simulink model "test_bu01_2018b"  (R2018b)
settings: Solver=FixedStepAuto  StartTime=0.0  StopTime=10  FixedStep=0.02  RelTol=1e-3
model workspace (MAT data in the model file):
  Ixx = 0.8
  Iyy = 2.075
  Izz = 1.25
  K = 0.75
  Mass = 11.5
  b = 0
libraries: simulink x10, aerolibutil x6, vrlib x4, sharedtransform x4, sharedutil x3, shared6dof x1
(part 4 of 4)

== system test_bu01_2018b/bu01_model/动力系统模型/Motor1_TM_P/TM1654P /螺旋桨模型/螺旋桨气动/计算螺旋桨气动系数/计算Ctz ==
  Miu : Inport
  Lumda : Inport  Port=2
  Add2 : Sum  Inputs=++-+-
  Add3 : Sum  Inputs=++-+
  Constant3 : Constant  Value=0.0651
  Constant4 : Constant  Value=0.0845
  Gain10 : Gain  Gain=0.0583
  Gain11 : Gain  Gain=0.3529
  Gain6 : Gain  Gain=0.0579
  Gain7 : Gain  Gain=0.0066
  Gain8 : Gain  Gain=-0.2325
  Gain9 : Gain  Gain=0.1346
  Lumda1 : InportShadow  Port=2
  Multiply2 : Product
  Square3 : Math  Operator=square  SaturateOnIntegerOverflow=on
  Square4 : Math  Operator=square  SaturateOnIntegerOverflow=on
  Square5 : Math  Operator=square  SaturateOnIntegerOverflow=on
  Ctz : Outport
  wires:
  Gain7/1 -> Add3/3
  Gain6/1 -> Add3/2
  Multiply2/1 -> Add3/4
  Add3/1 -> Ctz/1  "Ctz"
  Miu/1 -> Square4/1, Gain6/1, Square3/1, Gain8/1
  Lumda/1 -> Square5/1, Gain10/1
  Constant3/1 -> Add3/1
  Add2/1 -> Multiply2/2
  Square4/1 -> Gain9/1
  Constant4/1 -> Add2/3
  Gain9/1 -> Add2/2
  Square5/1 -> Gain11/1
  Gain11/1 -> Add2/5
  Gain8/1 -> Add2/1
  Square3/1 -> Gain7/1
  Gain10/1 -> Add2/4
  Lumda1/1 -> Multiply2/1

== system test_bu01_2018b/bu01_model/动力系统模型/Motor2_TM_N/TM1654N /螺旋桨模型/螺旋桨气动/计算螺旋桨气动系数/计算Cmx ==
  Miu : Inport
  Lumda : Inport  Port=2
  Add : Sum  Inputs=++--
  Constant : Constant  Value=0.0101
  Gain : Gain  Gain=0.0041
  Gain1 : Gain  Gain=0.009
  Gain2 : Gain  Gain=0.0032
  Multiply : Product
  Square : Math  Operator=square  SaturateOnIntegerOverflow=on
  Cmx : Outport
  wires:
  Multiply/1 -> Cmx/1  "Cmx"
  Lumda/1 -> Square/1, Gain1/1
  Gain2/1 -> Add/4
  Square/1 -> Gain2/1
  Gain/1 -> Add/2
  Constant/1 -> Add/1
  Miu/1 -> Multiply/1, Gain/1
  Gain1/1 -> Add/3
  Add/1 -> Multiply/2

== system test_bu01_2018b/bu01_model/动力系统模型/Motor2_TM_N/TM1654N /螺旋桨模型/螺旋桨气动/计算螺旋桨气动系数/计算Cmy ==
  Miu : Inport
  Lumda : Inport  Port=2
  Add1 : Sum  Inputs=++--
  Constant1 : Constant  Value=0.0101
  Gain1 : Gain  Gain=0.0041
  Gain3 : Gain  Gain=0.009
  Gain4 : Gain  Gain=0.0032
  Multiply1 : Product
  Square2 : Math  Operator=square  SaturateOnIntegerOverflow=on
  Cmy : Outport
  wires:
  Miu/1 -> Multiply1/1, Gain1/1
  Constant1/1 -> Add1/1
  Add1/1 -> Multiply1/2
  Gain4/1 -> Add1/4
  Square2/1 -> Gain4/1
  Lumda/1 -> Square2/1, Gain3/1
  Gain3/1 -> Add1/3
  Multiply1/1 -> Cmy/1  "Cmy"
  Gain1/1 -> Add1/2

== system test_bu01_2018b/bu01_model/动力系统模型/Motor2_TM_N/TM1654N /螺旋桨模型/螺旋桨气动/计算螺旋桨气动系数/计算Cmz ==
  Miu : Inport
  Lumda : Inport  Port=2
  Add2 : Sum  Inputs=+-+--
  Add3 : Sum  Inputs=+-++
  Constant3 : Constant  Value=0.0036
  Constant4 : Constant  Value=0.0023
  Gain10 : Gain  Gain=0.0105
  Gain11 : Gain  Gain=0.0078
  Gain6 : Gain  Gain=0.0006554
  Gain7 : Gain  Gain=0.00080732
  Gain8 : Gain  Gain=0.006
  Gain9 : Gain  Gain=0.0043
  Lumda1 : InportShadow  Port=2
  Multiply2 : Product
  Square3 : Math  Operator=square  SaturateOnIntegerOverflow=on
  Square4 : Math  Operator=square  SaturateOnIntegerOverflow=on
  Square5 : Math  Operator=square  SaturateOnIntegerOverflow=on
  Cmz : Outport
  wires:
  Lumda1/1 -> Multiply2/1
  Gain10/1 -> Add2/4
  Square3/1 -> Gain7/1
  Gain8/1 -> Add2/1
  Gain11/1 -> Add2/5
  Square5/1 -> Gain11/1
  Gain9/1 -> Add2/2
  Constant4/1 -> Add2/3
  Square4/1 -> Gain9/1
  Add2/1 -> Multiply2/2
  Constant3/1 -> Add3/1
  Lumda/1 -> Gain10/1, Square5/1
  Miu/1 -> Gain6/1, Square3/1, Square4/1, Gain8/1
  Add3/1 -> Cmz/1  "Cmz"
  Multiply2/1 -> Add3/4
  Gain6/1 -> Add3/2
  Gain7/1 -> Add3/3

== system test_bu01_2018b/bu01_model/动力系统模型/Motor2_TM_N/TM1654N /螺旋桨模型/螺旋桨气动/计算螺旋桨气动系数/计算Ctx ==
  Miu : Inport
  Lumda : Inport  Port=2
  Add : Sum  Inputs=++-+
  Constant : Constant  Value=-0.0074
  Gain : Gain  Gain=0.00051704
  Gain1 : Gain  Gain=0.0073
  Gain2 : Gain  Gain=0.018
  Multiply : Product
  Square : Math  Operator=square  SaturateOnIntegerOverflow=on
  Ctx : Outport
  wires:
  Add/1 -> Multiply/2
  Gain1/1 -> Add/3
  Miu/1 -> Multiply/1, Gain/1
  Constant/1 -> Add/1
  Gain/1 -> Add/2
  Square/1 -> Gain2/1
  Gain2/1 -> Add/4
  Lumda/1 -> Square/1, Gain1/1
  Multiply/1 -> Ctx/1  "Ctx"

== system test_bu01_2018b/bu01_model/动力系统模型/Motor2_TM_N/TM1654N /螺旋桨模型/螺旋桨气动/计算螺旋桨气动系数/计算Cty ==
  Miu : Inport
  Lumda : Inport  Port=2
  Add1 : Sum  Inputs=+++-
  Constant : Constant  Value=3
  Constant1 : Constant  Value=-0.002  OutDataTypeStr=double
  Gain3 : Gain  Gain=0.0103
  Gain4 : Gain  Gain=0.0168
  Gain5 : Gain  Gain=0.0897
  Multiply1 : Product
  Power : Math  Operator=pow  SaturateOnIntegerOverflow=on
  Square2 : Math  Operator=square  SaturateOnIntegerOverflow=on
  Cty : Outport
  wires:
  Gain5/1 -> Add1/4
  Multiply1/1 -> Cty/1  "Cty"
  Gain3/1 -> Add1/2
  Lumda/1 -> Power/1, Square2/1, Gain3/1
  Square2/1 -> Gain4/1
  Constant/1 -> Power/2
  Gain4/1 -> Add1/3
  Add1/1 -> Multiply1/2
  Constant1/1 -> Add1/1
  Power/1 -> Gain5/1
  Miu/1 -> Multiply1/1

== system test_bu01_2018b/bu01_model/动力系统模型/Motor2_TM_N/TM1654N /螺旋桨模型/螺旋桨气动/计算螺旋桨气动系数/计算Ctz ==
  Miu : Inport
  Lumda : Inport  Port=2
  Add2 : Sum  Inputs=++-+-
  Add3 : Sum  Inputs=++-+
  Constant3 : Constant  Value=0.0651
  Constant4 : Constant  Value=0.0845
  Gain10 : Gain  Gain=0.0583
  Gain11 : Gain  Gain=0.3529
  Gain6 : Gain  Gain=0.0579
  Gain7 : Gain  Gain=0.0066
  Gain8 : Gain  Gain=-0.2325
  Gain9 : Gain  Gain=0.1346
  Lumda1 : InportShadow  Port=2
  Multiply2 : Product
  Square3 : Math  Operator=square  SaturateOnIntegerOverflow=on
  Square4 : Math  Operator=square  SaturateOnIntegerOverflow=on
  Square5 : Math  Operator=square  SaturateOnIntegerOverflow=on
  Ctz : Outport
  wires:
  Gain7/1 -> Add3/3
  Gain6/1 -> Add3/2
  Multiply2/1 -> Add3/4
  Add3/1 -> Ctz/1  "Ctz"
  Miu/1 -> Gain8/1, Square4/1, Square3/1, Gain6/1
  Lumda/1 -> Square5/1, Gain10/1
  Constant3/1 -> Add3/1
  Add2/1 -> Multiply2/2
  Square4/1 -> Gain9/1
  Constant4/1 -> Add2/3
  Gain9/1 -> Add2/2
  Square5/1 -> Gain11/1
  Gain11/1 -> Add2/5
  Gain8/1 -> Add2/1
  Square3/1 -> Gain7/1
  Gain10/1 -> Add2/4
  Lumda1/1 -> Multiply2/1

== system test_bu01_2018b/bu01_model/动力系统模型/Motor3_TM_P/TM1654P /螺旋桨模型/螺旋桨气动/计算螺旋桨气动系数/计算Cmx ==
  Miu : Inport
  Lumda : Inport  Port=2
  Add : Sum  Inputs=++--
  Constant : Constant  Value=0.0101
  Gain : Gain  Gain=0.0041
  Gain1 : Gain  Gain=0.009
  Gain2 : Gain  Gain=0.0032
  Multiply : Product
  Square : Math  Operator=square  SaturateOnIntegerOverflow=on
  Cmx : Outport
  wires:
  Multiply/1 -> Cmx/1  "Cmx"
  Lumda/1 -> Square/1, Gain1/1
  Gain2/1 -> Add/4
  Square/1 -> Gain2/1
  Gain/1 -> Add/2
  Constant/1 -> Add/1
  Miu/1 -> Gain/1, Multiply/1
  Gain1/1 -> Add/3
  Add/1 -> Multiply/2

== system test_bu01_2018b/bu01_model/动力系统模型/Motor3_TM_P/TM1654P /螺旋桨模型/螺旋桨气动/计算螺旋桨气动系数/计算Cmy ==
  Miu : Inport
  Lumda : Inport  Port=2
  Add1 : Sum  Inputs=++++-
  Constant : Constant  Value=3
  Constant1 : Constant  Value=-0.015
  Gain1 : Gain  Gain=0.0115
  Gain2 : Gain  Gain=0.1908
  Gain3 : Gain  Gain=0.0146
  Gain4 : Gain  Gain=0.0484
  Multiply1 : Product
  Power : Math  Operator=pow  SaturateOnIntegerOverflow=on
  Square2 : Math  Operator=square  SaturateOnIntegerOverflow=on
  Cmy : Outport
  wires:
  Gain2/1 -> Add1/5
  Power/1 -> Gain2/1
  Constant/1 -> Power/2
  Miu/1 -> Multiply1/1, Gain1/1
  Constant1/1 -> Add1/1
  Add1/1 -> Multiply1/2
  Gain4/1 -> Add1/4
  Square2/1 -> Gain4/1
  Lumda/1 -> Square2/1, Power/1, Gain3/1
  Gain3/1 -> Add1/3
  Multiply1/1 -> Cmy/1  "Cmy"
  Gain1/1 -> Add1/2

== system test_bu01_2018b/bu01_model/动力系统模型/Motor3_TM_P/TM1654P /螺旋桨模型/螺旋桨气动/计算螺旋桨气动系数/计算Cmz ==
  Miu : Inport
  Lumda : Inport  Port=2
  Add2 : Sum  Inputs=+-+--
  Add3 : Sum  Inputs=+-++
  Constant3 : Constant  Value=0.0036
  Constant4 : Constant  Value=0.0023
  Gain10 : Gain  Gain=0.0105
  Gain11 : Gain  Gain=0.0078
  Gain6 : Gain  Gain=0.0006554
  Gain7 : Gain  Gain=0.00080732
  Gain8 : Gain  Gain=0.006
  Gain9 : Gain  Gain=0.0043
  Lumda1 : InportShadow  Port=2
  Multiply2 : Product
  Square3 : Math  Operator=square  SaturateOnIntegerOverflow=on
  Square4 : Math  Operator=square  SaturateOnIntegerOverflow=on
  Square5 : Math  Operator=square  SaturateOnIntegerOverflow=on
  Cmz : Outport
  wires:
  Lumda1/1 -> Multiply2/1
  Gain10/1 -> Add2/4
  Square3/1 -> Gain7/1
  Gain8/1 -> Add2/1
  Gain11/1 -> Add2/5
  Square5/1 -> Gain11/1
  Gain9/1 -> Add2/2
  Constant4/1 -> Add2/3
  Square4/1 -> Gain9/1
  Add2/1 -> Multiply2/2
  Constant3/1 -> Add3/1
  Lumda/1 -> Gain10/1, Square5/1
  Miu/1 -> Gain6/1, Square3/1, Square4/1, Gain8/1
  Add3/1 -> Cmz/1  "Cmz"
  Multiply2/1 -> Add3/4
  Gain6/1 -> Add3/2
  Gain7/1 -> Add3/3

== system test_bu01_2018b/bu01_model/动力系统模型/Motor3_TM_P/TM1654P /螺旋桨模型/螺旋桨气动/计算螺旋桨气动系数/计算Ctx ==
  Miu : Inport
  Lumda : Inport  Port=2
  Add : Sum  Inputs=++-+
  Constant : Constant  Value=-0.0074
  Gain : Gain  Gain=0.00051704
  Gain1 : Gain  Gain=0.0073
  Gain2 : Gain  Gain=0.018
  Multiply : Product
  Square : Math  Operator=square  SaturateOnIntegerOverflow=on
  Ctx : Outport
  wires:
  Add/1 -> Multiply/2
  Gain1/1 -> Add/3
  Miu/1 -> Multiply/1, Gain/1
  Constant/1 -> Add/1
  Gain/1 -> Add/2
  Square/1 -> Gain2/1
  Gain2/1 -> Add/4
  Lumda/1 -> Square/1, Gain1/1
  Multiply/1 -> Ctx/1  "Ctx"

== system test_bu01_2018b/bu01_model/动力系统模型/Motor3_TM_P/TM1654P /螺旋桨模型/螺旋桨气动/计算螺旋桨气动系数/计算Cty ==
  Miu : Inport
  Lumda : Inport  Port=2
  Add1 : Sum  Inputs=+++-
  Constant : Constant  Value=3
  Constant1 : Constant  Value=-0.002  OutDataTypeStr=double
  Gain3 : Gain  Gain=0.0103
  Gain4 : Gain  Gain=0.0168
  Gain5 : Gain  Gain=0.0897
  Multiply1 : Product
  Power : Math  Operator=pow  SaturateOnIntegerOverflow=on
  Square2 : Math  Operator=square  SaturateOnIntegerOverflow=on
  Cty : Outport
  wires:
  Gain5/1 -> Add1/4
  Multiply1/1 -> Cty/1  "Cty"
  Gain3/1 -> Add1/2
  Lumda/1 -> Power/1, Square2/1, Gain3/1
  Square2/1 -> Gain4/1
  Constant/1 -> Power/2
  Gain4/1 -> Add1/3
  Add1/1 -> Multiply1/2
  Constant1/1 -> Add1/1
  Power/1 -> Gain5/1
  Miu/1 -> Multiply1/1

== system test_bu01_2018b/bu01_model/动力系统模型/Motor3_TM_P/TM1654P /螺旋桨模型/螺旋桨气动/计算螺旋桨气动系数/计算Ctz ==
  Miu : Inport
  Lumda : Inport  Port=2
  Add2 : Sum  Inputs=++-+-
  Add3 : Sum  Inputs=++-+
  Constant3 : Constant  Value=0.0651
  Constant4 : Constant  Value=0.0845
  Gain10 : Gain  Gain=0.0583
  Gain11 : Gain  Gain=0.3529
  Gain6 : Gain  Gain=0.0579
  Gain7 : Gain  Gain=0.0066
  Gain8 : Gain  Gain=-0.2325
  Gain9 : Gain  Gain=0.1346
  Lumda1 : InportShadow  Port=2
  Multiply2 : Product
  Square3 : Math  Operator=square  SaturateOnIntegerOverflow=on
  Square4 : Math  Operator=square  SaturateOnIntegerOverflow=on
  Square5 : Math  Operator=square  SaturateOnIntegerOverflow=on
  Ctz : Outport
  wires:
  Gain7/1 -> Add3/3
  Gain6/1 -> Add3/2
  Multiply2/1 -> Add3/4
  Add3/1 -> Ctz/1  "Ctz"
  Miu/1 -> Square4/1, Gain6/1, Square3/1, Gain8/1
  Lumda/1 -> Square5/1, Gain10/1
  Constant3/1 -> Add3/1
  Add2/1 -> Multiply2/2
  Square4/1 -> Gain9/1
  Constant4/1 -> Add2/3
  Gain9/1 -> Add2/2
  Square5/1 -> Gain11/1
  Gain11/1 -> Add2/5
  Gain8/1 -> Add2/1
  Square3/1 -> Gain7/1
  Gain10/1 -> Add2/4
  Lumda1/1 -> Multiply2/1

== system test_bu01_2018b/bu01_model/动力系统模型/Motor4_TM_N/TM1654N /螺旋桨模型/螺旋桨气动/计算螺旋桨气动系数/计算Cmx ==
  Miu : Inport
  Lumda : Inport  Port=2
  Add : Sum  Inputs=++--
  Constant : Constant  Value=0.0101
  Gain : Gain  Gain=0.0041
  Gain1 : Gain  Gain=0.009
  Gain2 : Gain  Gain=0.0032
  Multiply : Product
  Square : Math  Operator=square  SaturateOnIntegerOverflow=on
  Cmx : Outport
  wires:
  Multiply/1 -> Cmx/1  "Cmx"
  Lumda/1 -> Square/1, Gain1/1
  Gain2/1 -> Add/4
  Square/1 -> Gain2/1
  Gain/1 -> Add/2
  Constant/1 -> Add/1
  Miu/1 -> Multiply/1, Gain/1
  Gain1/1 -> Add/3
  Add/1 -> Multiply/2

== system test_bu01_2018b/bu01_model/动力系统模型/Motor4_TM_N/TM1654N /螺旋桨模型/螺旋桨气动/计算螺旋桨气动系数/计算Cmy ==
  Miu : Inport
  Lumda : Inport  Port=2
  Add1 : Sum  Inputs=++--
  Constant1 : Constant  Value=0.0101
  Gain1 : Gain  Gain=0.0041
  Gain3 : Gain  Gain=0.009
  Gain4 : Gain  Gain=0.0032
  Multiply1 : Product
  Square2 : Math  Operator=square  SaturateOnIntegerOverflow=on
  Cmy : Outport
  wires:
  Miu/1 -> Multiply1/1, Gain1/1
  Constant1/1 -> Add1/1
  Add1/1 -> Multiply1/2
  Gain4/1 -> Add1/4
  Square2/1 -> Gain4/1
  Lumda/1 -> Square2/1, Gain3/1
  Gain3/1 -> Add1/3
  Multiply1/1 -> Cmy/1  "Cmy"
  Gain1/1 -> Add1/2

== system test_bu01_2018b/bu01_model/动力系统模型/Motor4_TM_N/TM1654N /螺旋桨模型/螺旋桨气动/计算螺旋桨气动系数/计算Cmz ==
  Miu : Inport
  Lumda : Inport  Port=2
  Add2 : Sum  Inputs=+-+--
  Add3 : Sum  Inputs=+-++
  Constant3 : Constant  Value=0.0036
  Constant4 : Constant  Value=0.0023
  Gain10 : Gain  Gain=0.0105
  Gain11 : Gain  Gain=0.0078
  Gain6 : Gain  Gain=0.0006554
  Gain7 : Gain  Gain=0.00080732
  Gain8 : Gain  Gain=0.006
  Gain9 : Gain  Gain=0.0043
  Lumda1 : InportShadow  Port=2
  Multiply2 : Product
  Square3 : Math  Operator=square  SaturateOnIntegerOverflow=on
  Square4 : Math  Operator=square  SaturateOnIntegerOverflow=on
  Square5 : Math  Operator=square  SaturateOnIntegerOverflow=on
  Cmz : Outport
  wires:
  Lumda1/1 -> Multiply2/1
  Gain10/1 -> Add2/4
  Square3/1 -> Gain7/1
  Gain8/1 -> Add2/1
  Gain11/1 -> Add2/5
  Square5/1 -> Gain11/1
  Gain9/1 -> Add2/2
  Constant4/1 -> Add2/3
  Square4/1 -> Gain9/1
  Add2/1 -> Multiply2/2
  Constant3/1 -> Add3/1
  Lumda/1 -> Gain10/1, Square5/1
  Miu/1 -> Gain6/1, Square3/1, Square4/1, Gain8/1
  Add3/1 -> Cmz/1  "Cmz"
  Multiply2/1 -> Add3/4
  Gain6/1 -> Add3/2
  Gain7/1 -> Add3/3

== system test_bu01_2018b/bu01_model/动力系统模型/Motor4_TM_N/TM1654N /螺旋桨模型/螺旋桨气动/计算螺旋桨气动系数/计算Ctx ==
  Miu : Inport
  Lumda : Inport  Port=2
  Add : Sum  Inputs=++-+
  Constant : Constant  Value=-0.0074
  Gain : Gain  Gain=0.00051704
  Gain1 : Gain  Gain=0.0073
  Gain2 : Gain  Gain=0.018
  Multiply : Product
  Square : Math  Operator=square  SaturateOnIntegerOverflow=on
  Ctx : Outport
  wires:
  Add/1 -> Multiply/2
  Gain1/1 -> Add/3
  Miu/1 -> Multiply/1, Gain/1
  Constant/1 -> Add/1
  Gain/1 -> Add/2
  Square/1 -> Gain2/1
  Gain2/1 -> Add/4
  Lumda/1 -> Square/1, Gain1/1
  Multiply/1 -> Ctx/1  "Ctx"

== system test_bu01_2018b/bu01_model/动力系统模型/Motor4_TM_N/TM1654N /螺旋桨模型/螺旋桨气动/计算螺旋桨气动系数/计算Cty ==
  Miu : Inport
  Lumda : Inport  Port=2
  Add1 : Sum  Inputs=+++-
  Constant : Constant  Value=3
  Constant1 : Constant  Value=-0.002  OutDataTypeStr=double
  Gain3 : Gain  Gain=0.0103
  Gain4 : Gain  Gain=0.0168
  Gain5 : Gain  Gain=0.0897
  Multiply1 : Product
  Power : Math  Operator=pow  SaturateOnIntegerOverflow=on
  Square2 : Math  Operator=square  SaturateOnIntegerOverflow=on
  Cty : Outport
  wires:
  Gain5/1 -> Add1/4
  Multiply1/1 -> Cty/1  "Cty"
  Gain3/1 -> Add1/2
  Lumda/1 -> Power/1, Square2/1, Gain3/1
  Square2/1 -> Gain4/1
  Constant/1 -> Power/2
  Gain4/1 -> Add1/3
  Add1/1 -> Multiply1/2
  Constant1/1 -> Add1/1
  Power/1 -> Gain5/1
  Miu/1 -> Multiply1/1

== system test_bu01_2018b/bu01_model/动力系统模型/Motor4_TM_N/TM1654N /螺旋桨模型/螺旋桨气动/计算螺旋桨气动系数/计算Ctz ==
  Miu : Inport
  Lumda : Inport  Port=2
  Add2 : Sum  Inputs=++-+-
  Add3 : Sum  Inputs=++-+
  Constant3 : Constant  Value=0.0651
  Constant4 : Constant  Value=0.0845
  Gain10 : Gain  Gain=0.0583
  Gain11 : Gain  Gain=0.3529
  Gain6 : Gain  Gain=0.0579
  Gain7 : Gain  Gain=0.0066
  Gain8 : Gain  Gain=-0.2325
  Gain9 : Gain  Gain=0.1346
  Lumda1 : InportShadow  Port=2
  Multiply2 : Product
  Square3 : Math  Operator=square  SaturateOnIntegerOverflow=on
  Square4 : Math  Operator=square  SaturateOnIntegerOverflow=on
  Square5 : Math  Operator=square  SaturateOnIntegerOverflow=on
  Ctz : Outport
  wires:
  Gain7/1 -> Add3/3
  Gain6/1 -> Add3/2
  Multiply2/1 -> Add3/4
  Add3/1 -> Ctz/1  "Ctz"
  Miu/1 -> Gain8/1, Square4/1, Square3/1, Gain6/1
  Lumda/1 -> Square5/1, Gain10/1
  Constant3/1 -> Add3/1
  Add2/1 -> Multiply2/2
  Square4/1 -> Gain9/1
  Constant4/1 -> Add2/3
  Gain9/1 -> Add2/2
  Square5/1 -> Gain11/1
  Gain11/1 -> Add2/5
  Gain8/1 -> Add2/1
  Square3/1 -> Gain7/1
  Gain10/1 -> Add2/4
  Lumda1/1 -> Multiply2/1

== matlab function test_bu01_2018b/角度控制器/求取航向衰减后的期望四元数/MATLAB Function ==
  data: src input; q output; dst input
function q = vec2quat(src, dst)
    quat = [1 0 0 0];
    cr = cross(src, dst);
    dt = dot(src, dst);
    % 处理向量夹角为180度的情况
    if norm(cr) < eps && dt < 0
       cr = abs(src);
       if cr(1) < cr(2)
          if cr(1) < cr(3)
              cr = [1 0 0];
          else
              cr = [0 0 1];
          end
       else
           if cr(2) < cr(3)
               cr = [0 1 0];
           else
               cr = [0 0 1];
           end
       end
       quat(1) = 0;
       cr = cross(src, cr);
    else
        quat(1) = dt + norm(src)*norm(dst);
    end
    quat(2) = cr(1);
    quat(3) = cr(2);
    quat(4) = cr(3);
    q = quat;
